simulink model "testoccplot"  (R2014a)
settings: Solver=ode45  StartTime=0.0  StopTime=10.0  RelTol=1e-3
values from neighbouring files (symbols this model uses):
  occVec = [size(occ)';occBox';reshape(occ,numel(occ),1)]    [mapproc.m]
settings Model: Creator=aeagr  LastModifiedBy=aeagr

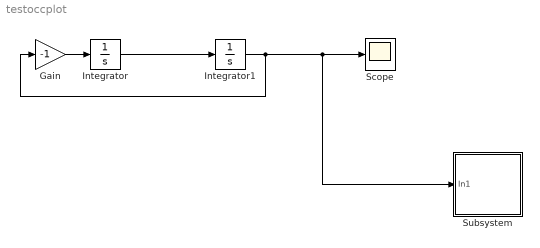
== system testoccplot ==
  Gain : Gain  Gain=-1
  Integrator : Integrator
  Integrator1 : Integrator  InitialCondition=1
  Scope : Scope
  Subsystem : Subsystem  TreatAsAtomicUnit=on  SystemSampleTime=0.1
  wires:
  Integrator/1 -> Integrator1/1
  Gain/1 -> Integrator/1
  Integrator1/1 -> Subsystem/1(In1), Scope/1, Gain/1

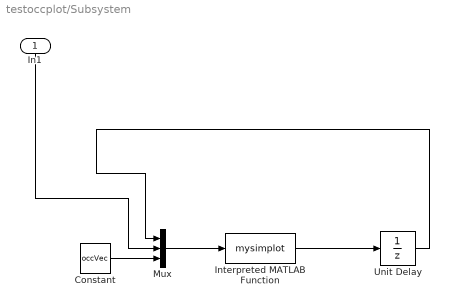
== system testoccplot/Subsystem ==
  In1 : Inport
  Constant : Constant  Value=occVec
  Interpreted MATLAB Function : MATLABFcn  MATLABFcn=mysimplot  OutputDimensions=1
  Mux : Mux  Inputs=3
  Unit Delay : UnitDelay  SampleTime=-1
  wires:
  In1/1 -> Mux/2
  Interpreted MATLAB Function/1 -> Unit Delay/1
  Unit Delay/1 -> Mux/1
  Mux/1 -> Interpreted MATLAB Function/1
  Constant/1 -> Mux/3
